simulink model "RUNES_demo"  (Simulink 7.4)
settings: Solver=ode45  StartTime=0.0  StopTime=inf  RelTol=1e-3
InitFcn:
  | init
values from neighbouring files (symbols this model uses):
  D = 30    [init.m]
  nbrOfMotes = 3    [init.m]
  R1 = 3    [init.m]
  R2 = 3    [init.m]
  trackLength = 800    [init.m]
  trackWidth = 200    [init.m]
undefined symbols (not defined in the file or in its folder): nodeXpos, nodeYpos, WLAN
libraries: truetime x14, simulink x6
settings Model: Creator=anton  LastModifiedBy=anton  ExtModeAutoUpdateStatusClock=off
settings DataIOCC: LimitDataPoints=off  SaveOutput=off  SaveTime=off
settings OptimizationCC: BooleanDataType=off
settings DebuggingCC: SaveWithParameterizedLinksMsg=none  SignalResolutionControl=TryResolveAllWithWarning  SolverPrmCheckMsg=none  MultiTaskDSMMsg=warning  MultiTaskCondExecSysMsg=none  UnconnectedInputMsg=none  UnconnectedOutputMsg=none  UnconnectedLineMsg=none  StrictBusMsg=None
settings HardwareCC: TargetUnknown=on
settings RTWCC: IncludeERTFirstTime=on

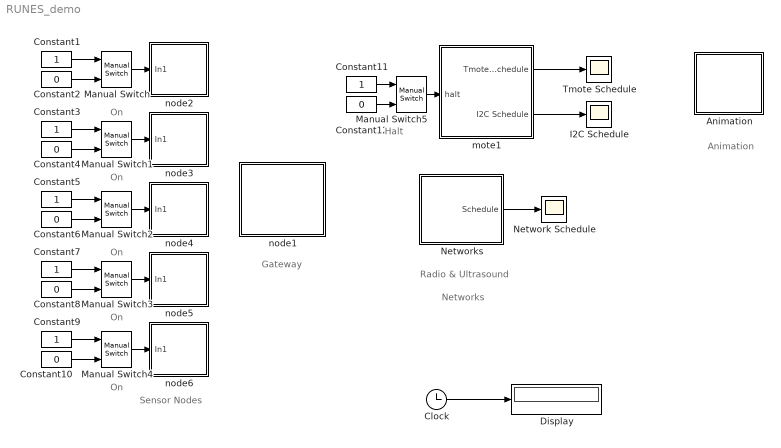
== system RUNES_demo ==
  note: Sensor Nodes
  note: Gateway
  note: Radio & Ultrasound
  note: Networks
  note: On
  note: On
  note: On
  note: On
  note: On
  note: Animation
  note: Halt
  Animation : Subsystem
  Clock : Clock
      settings: Decimation=10
  Constant{1,3,5,7,9,11} (6 alike) : Constant
  Constant{2,4,6,8,10,12} (6 alike) : Constant  Value=0
  Display : Display
  I2C Schedule : Scope
      settings: TimeRange=5  YMin=1  YMax=5.5  SaveName=nschedule1
  Manual Switch{,1..5} (6 alike) : simulink/Signal Routing/Manual Switch  SystemSampleTime=-1  sw=1  action=0  varsize=off
  Network Schedule : Scope
      settings: TimeRange=5  YMin=1  YMax=9  SaveName=nschedule
  Networks : Subsystem
  Tmote Schedule : Scope
      settings: TimeRange=5  YMin=1  YMax=9  SaveName=nschedule2
  mote1 : Subsystem  mask{moteNbr=1}
      mask Display: image(imread('RBBot.jpg'))
  node1 : Subsystem  mask{nodeNbr=1}
      mask init:
      | set_param(strcat(gcb,'/Goto'),'GotoTag',strcat('node',num2str(nodeNbr)));
      | set_param(strcat(gcb,'/X'),'Value',strcat('nodeXpos(',strcat(num2str(nodeNbr), ')')));
      | set_param(strcat(gcb,'/Y'),'Value',strcat('nodeYpos(',strcat(num2str(nodeNbr), ')')));
      mask Display: image(imread('gateway.jpg'))
  node2 : Subsystem  mask{nodeNbr=2}
      mask init: same as RUNES_demo/node1
      mask Display: image(imread('mote.jpg'))
  node3 : Subsystem  mask{nodeNbr=3}
      mask init: same as RUNES_demo/node1
      mask Display: image(imread('mote.jpg'))
  node4 : Subsystem  mask{nodeNbr=4}
      mask init: same as RUNES_demo/node1
      mask Display: image(imread('mote.jpg'))
  node5 : Subsystem  mask{nodeNbr=5}
      mask init: same as RUNES_demo/node1
      mask Display: image(imread('mote.jpg'))
  node6 : Subsystem  mask{nodeNbr=6}
      mask init: same as RUNES_demo/node1
      mask Display: image(imread('mote.jpg'))
  wires:
  Constant1/1 -> Manual Switch/1
  Constant2/1 -> Manual Switch/2
  Constant3/1 -> Manual Switch1/1
  Constant4/1 -> Manual Switch1/2
  Constant5/1 -> Manual Switch2/1
  Constant6/1 -> Manual Switch2/2
  Constant7/1 -> Manual Switch3/1
  Constant8/1 -> Manual Switch3/2
  Constant9/1 -> Manual Switch4/1
  Constant10/1 -> Manual Switch4/2
  Manual Switch/1 -> node2/1(In1)
  Manual Switch3/1 -> node5/1(In1)
  Manual Switch4/1 -> node6/1(In1)
  Manual Switch1/1 -> node3/1(In1)
  Networks/1(Schedule) -> Network Schedule/1
  Constant11/1 -> Manual Switch5/1
  Constant12/1 -> Manual Switch5/2
  Manual Switch5/1 -> mote1/1(halt)
  mote1/1(Tmote Schedule) -> Tmote Schedule/1
  mote1/2(I2C Schedule) -> I2C Schedule/1
  Clock/1 -> Display/1
  Manual Switch2/1 -> node4/1(In1)

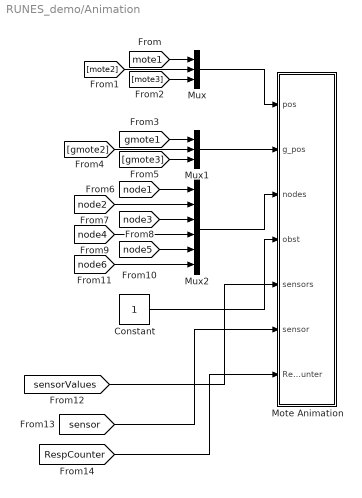
== system RUNES_demo/Animation ==
  Constant : Constant
  Mote Animation : Subsystem  mask{numMotes=nbrOfMotes, xmax=trackLength, ymax=trackWidth, ts=0.1}
      mask prompts: numMotes "Number of Motes"; ts "Update period"
  Mux : Mux  Inputs=[3 3 3]
  Mux1 : Mux  Inputs=[3 3 3]
  Mux2 : Mux  Inputs=6
  wires:
  Mux/1 -> Mote Animation/1(pos)
  [mote1] -> Mux/1
  [mote2] -> Mux/2
  [mote3] -> Mux/3
  Mux1/1 -> Mote Animation/2(g_pos)
  [gmote1] -> Mux1/1
  [gmote2] -> Mux1/2
  [gmote3] -> Mux1/3
  Constant/1 -> Mote Animation/4(obst)
  Mux2/1 -> Mote Animation/3(nodes)
  [node1] -> Mux2/1
  [node2] -> Mux2/2
  [node3] -> Mux2/3
  [node4] -> Mux2/4
  [node5] -> Mux2/5
  [node6] -> Mux2/6
  [sensorValues] -> Mote Animation/5(sensors)
  [sensor] -> Mote Animation/6(sensor)
  [RespCounter] -> Mote Animation/7(RespCounter)

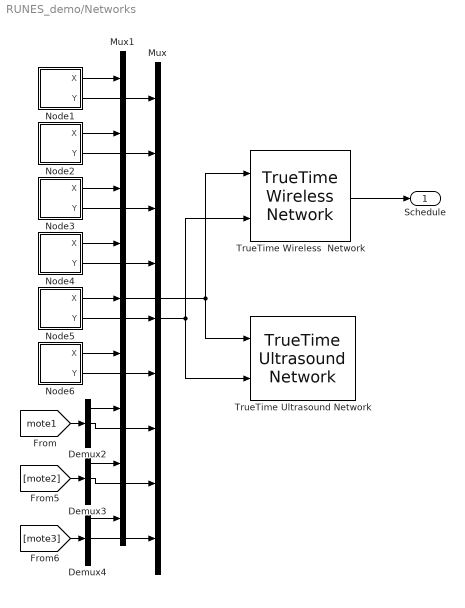
== system RUNES_demo/Networks ==
  Demux2 : Demux  Outputs=3
  Demux3 : Demux  Outputs=3
  Demux4 : Demux  Outputs=3
  Mux : Mux  Inputs=9
  Mux1 : Mux  Inputs=9
  Node1 : Subsystem  mask{nodeNbr=1}
      mask init:
      | set_param(strcat(gcb,'/From'),'GotoTag',strcat('node',num2str(nodeNbr)));
  Node2 : Subsystem  mask{nodeNbr=2}
      mask init:
      | set_param(strcat(gcb,'/From'),'GotoTag',strcat('node',num2str(nodeNbr)));
  Node3 : Subsystem  mask{nodeNbr=3}
      mask init:
      | set_param(strcat(gcb,'/From'),'GotoTag',strcat('node',num2str(nodeNbr)));
  Node4 : Subsystem  mask{nodeNbr=4}
      mask init:
      | set_param(strcat(gcb,'/From'),'GotoTag',strcat('node',num2str(nodeNbr)));
  Node5 : Subsystem  mask{nodeNbr=5}
      mask init:
      | set_param(strcat(gcb,'/From'),'GotoTag',strcat('node',num2str(nodeNbr)));
  Node6 : Subsystem  mask{nodeNbr=6}
      mask init:
      | set_param(strcat(gcb,'/From'),'GotoTag',strcat('node',num2str(nodeNbr)));
  TrueTime Ultrasound Network : truetime/TrueTime Ultrasound Network  SystemSampleTime=-1  nwnbr=2  nnodes=9  reach=260  pinglength=0.0  speedofsound=34400.0  scheduleoutput=off
  TrueTime Wireless  Network : truetime/TrueTime Wireless  Network  SystemSampleTime=-1  nwtype=802.11b (WLAN)  nwnbr=1  nnodes=9  rate=250000  minsize=248  transpower=transmitPower  threshold=receiverThreshold  use_pathloss_function=default  pathloss=pathloss  acktimeout=0.000864  retrylimit=3  error_threshold=errorCodingThreshold  lossprob=0  seed=0  scheduleoutput=on  poweroutput=off
  Schedule : Outport
  wires:
  Node1/1(X) -> Mux1/1
  Node2/1(X) -> Mux1/2
  Node3/1(X) -> Mux1/3
  Node4/1(X) -> Mux1/4
  Node5/1(X) -> Mux1/5
  Node6/1(X) -> Mux1/6
  Node6/2(Y) -> Mux/6
  Node5/2(Y) -> Mux/5
  Node4/2(Y) -> Mux/4
  Node3/2(Y) -> Mux/3
  Node2/2(Y) -> Mux/2
  Node1/2(Y) -> Mux/1
  [mote1] -> Demux2/1
  Demux2/1 -> Mux1/7
  [mote2] -> Demux3/1
  Demux3/1 -> Mux1/8
  Demux3/2 -> Mux/8
  Demux2/2 -> Mux/7
  [mote3] -> Demux4/1
  Demux4/1 -> Mux1/9
  Demux4/2 -> Mux/9
  Mux1/1 -> TrueTime Wireless  Network/1, TrueTime Ultrasound Network/1
  Mux/1 -> TrueTime Ultrasound Network/2, TrueTime Wireless  Network/2
  TrueTime Wireless  Network/1 -> Schedule/1

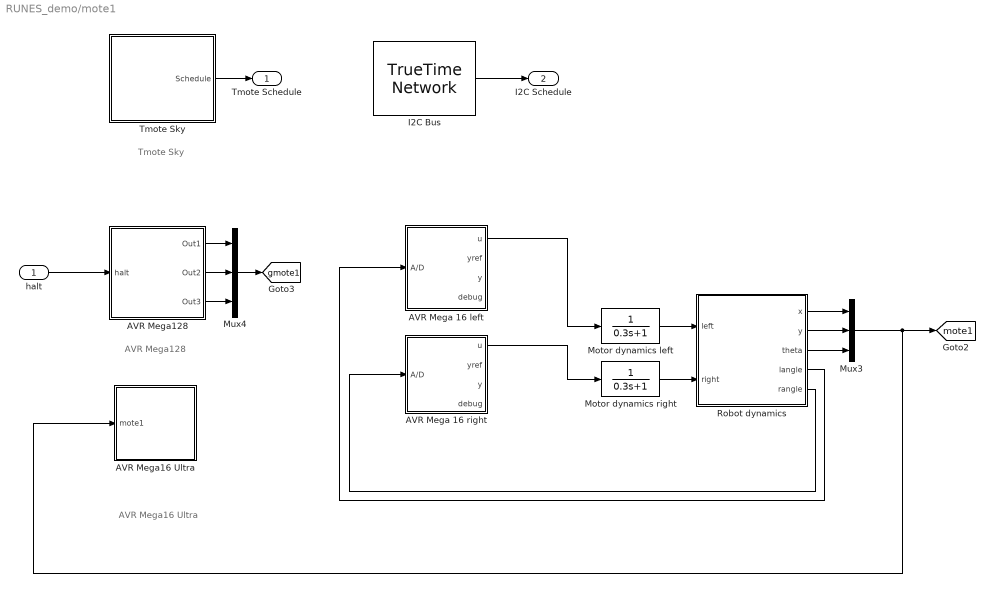
== system RUNES_demo/mote1 ==
  note: Tmote Sky
  note: AVR Mega16 Ultra
  note: AVR Mega128
  halt : Inport
  AVR Mega 16 left : Subsystem
      mask Display: image(imread('mega16.jpg'))
  AVR Mega 16 right : Subsystem
      mask Display: image(imread('mega16.jpg'))
  AVR Mega128 : Subsystem
      mask Display: image(imread('mega128.jpg'))
  AVR Mega16 Ultra : Subsystem
      mask Display: image(imread('mega16.jpg'))
  I2C Bus : truetime/TrueTime Network  SystemSampleTime=-1  nwtype=CSMA/CD (Ethernet)  nwnbr=3  nnodes=5  rate=10000000  minsize=512  lossprob=0  seed=0  bandwidths=[0.5 0.5]  slotsize=512  schedule=[1 1 2]  memsize=80000  buftype=Common buffer  overflow=Retransmit  dynSchedule=0  miniSlotSize=0  NIT=0  QSortMode=FIFO  sync=0  irtSchedule=0  nrtLength=0  nodeGraph=0  scheduleoutput=on
  Motor dynamics left : TransferFcn  Denominator=[0.3 1]
  Motor dynamics right : TransferFcn  Denominator=[0.3 1]
  Mux3 : Mux  Inputs=3
  Mux4 : Mux  Inputs=3
  Robot dynamics : Subsystem  TreatAsAtomicUnit=on
      mask Display: image(imread('model.png'))
  Tmote Sky : Subsystem
      mask Display: image(imread('Tmote.jpg'))
  Tmote Schedule : Outport
  I2C Schedule : Outport  Port=2
  tag scope: gmote1=global, mote1=global
  wires:
  Tmote Sky/1(Schedule) -> Tmote Schedule/1
  I2C Bus/1 -> I2C Schedule/1
  Mux4/1 -> [gmote1]
  halt/1 -> AVR Mega128/1(halt)
  Robot dynamics/4(langle) -> AVR Mega 16 left/1(A/D)
  Robot dynamics/5(rangle) -> AVR Mega 16 right/1(A/D)
  Motor dynamics right/1 -> Robot dynamics/2(right)
  Motor dynamics left/1 -> Robot dynamics/1(left)
  AVR Mega 16 left/1(u) -> Motor dynamics left/1
  AVR Mega 16 right/1(u) -> Motor dynamics right/1
  AVR Mega128/3(Out3) -> Mux4/3
  AVR Mega128/2(Out2) -> Mux4/2
  AVR Mega128/1(Out1) -> Mux4/1
  Robot dynamics/1(x) -> Mux3/1
  Robot dynamics/2(y) -> Mux3/2
  Robot dynamics/3(theta) -> Mux3/3
  Mux3/1 -> [mote1], AVR Mega16 Ultra/1(mote1)

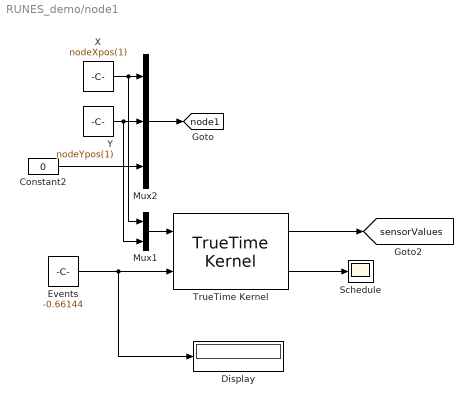
== system RUNES_demo/node1 ==
  Constant2 : Constant  Value=0
  Display : Display
  Events : Constant  Value=-0.66144
  Mux1 : Mux  Inputs=2
  Mux2 : Mux  Inputs=3
  Schedule : Scope
      settings: TickLabels=on  TimeRange=3.5  YMin=0  YMax=9.5  DataFormat=Array
  TrueTime Kernel : truetime/TrueTime Kernel  SystemSampleTime=-1  sfun=node_init  args=nodeNbr  ninputsoutputs=[2 5]  ntriggers=1  trigtype=falling  nwnodenbr=[1 nodeNbr; 2 nodeNbr]  clockoffsetdrift=[0 0]  schedoutput=on  battery=off  poweroutput=off  label=1: 1\n2: 1
  X : Constant  Value=nodeXpos(1)
  Y : Constant  Value=nodeYpos(1)
  tag scope: node1=global, sensorValues=global
  wires:
  X/1 -> Mux2/1, Mux1/1
  Y/1 -> Mux2/2, Mux1/2
  Mux2/1 -> [node1]
  Constant2/1 -> Mux2/3
  TrueTime Kernel/1 -> [sensorValues]
  Mux1/1 -> TrueTime Kernel/1
  TrueTime Kernel/2 -> Schedule/1
  Events/1 -> Display/1, TrueTime Kernel/2

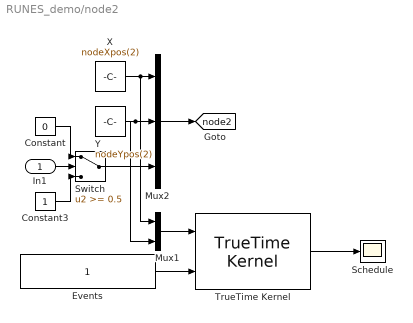
== system RUNES_demo/node2 ==
  In1 : Inport
  Constant : Constant  Value=0
  Constant3 : Constant
  Events : Constant
  Mux1 : Mux  Inputs=2
  Mux2 : Mux  Inputs=3
  Schedule : Scope
      settings: TickLabels=on  TimeRange=3.5  YMin=1.8  YMax=3.7  DataFormat=Array
  Switch : Switch  Threshold=0.5  SaturateOnIntegerOverflow=on  InputSameDT=on
  TrueTime Kernel : truetime/TrueTime Kernel  SystemSampleTime=-1  sfun=node_init  args=nodeNbr  ninputsoutputs=[2 0]  ntriggers=1  trigtype=either  nwnodenbr=[1 nodeNbr; 2 nodeNbr]  clockoffsetdrift=[0 0]  schedoutput=on  battery=off  poweroutput=off  label=1: 2\n2: 2
  X : Constant  Value=nodeXpos(2)
  Y : Constant  Value=nodeYpos(2)
  tag scope: node2=global
  wires:
  TrueTime Kernel/1 -> Schedule/1
  Events/1 -> TrueTime Kernel/2
  Mux2/1 -> [node2]
  Switch/1 -> Mux2/3
  Y/1 -> Mux1/2, Mux2/2
  X/1 -> Mux1/1, Mux2/1
  In1/1 -> Switch/2
  Constant3/1 -> Switch/3
  Constant/1 -> Switch/1
  Mux1/1 -> TrueTime Kernel/1

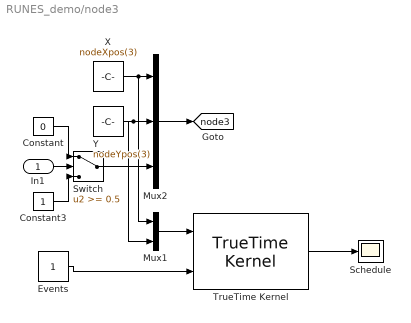
== system RUNES_demo/node3 ==
  In1 : Inport
  Constant : Constant  Value=0
  Constant3 : Constant
  Events : Constant
  Mux1 : Mux  Inputs=2
  Mux2 : Mux  Inputs=3
  Schedule : Scope
      settings: TickLabels=on  TimeRange=3.5  YMin=1.8  YMax=3.7  DataFormat=Array
  Switch : Switch  Threshold=0.5  SaturateOnIntegerOverflow=on  InputSameDT=on
  TrueTime Kernel : truetime/TrueTime Kernel  SystemSampleTime=-1  sfun=node_init  args=nodeNbr  ninputsoutputs=[2 0]  ntriggers=1  trigtype=either  nwnodenbr=[1 nodeNbr; 2 nodeNbr]  clockoffsetdrift=[0 0]  schedoutput=on  battery=off  poweroutput=off  label=1: 3\n2: 3
  X : Constant  Value=nodeXpos(3)
  Y : Constant  Value=nodeYpos(3)
  tag scope: node3=global
  wires:
  Mux1/1 -> TrueTime Kernel/1
  Constant/1 -> Switch/1
  Constant3/1 -> Switch/3
  In1/1 -> Switch/2
  X/1 -> Mux2/1, Mux1/1
  Y/1 -> Mux2/2, Mux1/2
  Switch/1 -> Mux2/3
  Mux2/1 -> [node3]
  Events/1 -> TrueTime Kernel/2
  TrueTime Kernel/1 -> Schedule/1

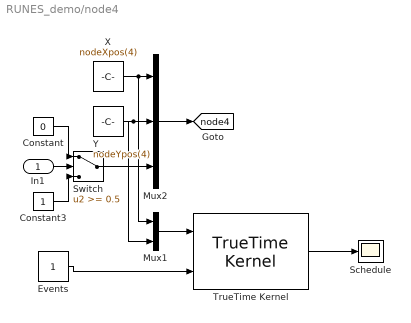
== system RUNES_demo/node4 ==
  In1 : Inport
  Constant : Constant  Value=0
  Constant3 : Constant
  Events : Constant
  Mux1 : Mux  Inputs=2
  Mux2 : Mux  Inputs=3
  Schedule : Scope
      settings: TickLabels=on  TimeRange=3.5  YMin=1.8  YMax=3.7  DataFormat=Array
  Switch : Switch  Threshold=0.5  SaturateOnIntegerOverflow=on  InputSameDT=on
  TrueTime Kernel : truetime/TrueTime Kernel  SystemSampleTime=-1  sfun=node_init  args=nodeNbr  ninputsoutputs=[2 0]  ntriggers=1  trigtype=either  nwnodenbr=[1 nodeNbr; 2 nodeNbr]  clockoffsetdrift=[0 0]  schedoutput=on  battery=off  poweroutput=off  label=1: 4\n2: 4
  X : Constant  Value=nodeXpos(4)
  Y : Constant  Value=nodeYpos(4)
  tag scope: node4=global
  wires:
  TrueTime Kernel/1 -> Schedule/1
  Events/1 -> TrueTime Kernel/2
  Mux2/1 -> [node4]
  Switch/1 -> Mux2/3
  Y/1 -> Mux1/2, Mux2/2
  X/1 -> Mux1/1, Mux2/1
  In1/1 -> Switch/2
  Constant3/1 -> Switch/3
  Constant/1 -> Switch/1
  Mux1/1 -> TrueTime Kernel/1

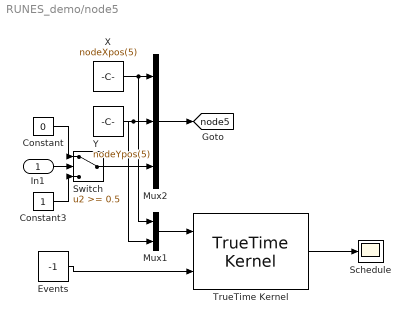
== system RUNES_demo/node5 ==
  In1 : Inport
  Constant : Constant  Value=0
  Constant3 : Constant
  Events : Constant  Value=-1
  Mux1 : Mux  Inputs=2
  Mux2 : Mux  Inputs=3
  Schedule : Scope
      settings: TickLabels=on  TimeRange=3.5  YMin=1.8  YMax=3.7  DataFormat=Array
  Switch : Switch  Threshold=0.5  SaturateOnIntegerOverflow=on  InputSameDT=on
  TrueTime Kernel : truetime/TrueTime Kernel  SystemSampleTime=-1  sfun=node_init  args=nodeNbr  ninputsoutputs=[2 0]  ntriggers=1  trigtype=either  nwnodenbr=[1 nodeNbr; 2 nodeNbr]  clockoffsetdrift=[0 0]  schedoutput=on  battery=off  poweroutput=off  label=1: 5\n2: 5
  X : Constant  Value=nodeXpos(5)
  Y : Constant  Value=nodeYpos(5)
  tag scope: node5=global
  wires:
  Mux1/1 -> TrueTime Kernel/1
  Constant/1 -> Switch/1
  Constant3/1 -> Switch/3
  In1/1 -> Switch/2
  X/1 -> Mux2/1, Mux1/1
  Y/1 -> Mux2/2, Mux1/2
  Switch/1 -> Mux2/3
  Mux2/1 -> [node5]
  Events/1 -> TrueTime Kernel/2
  TrueTime Kernel/1 -> Schedule/1

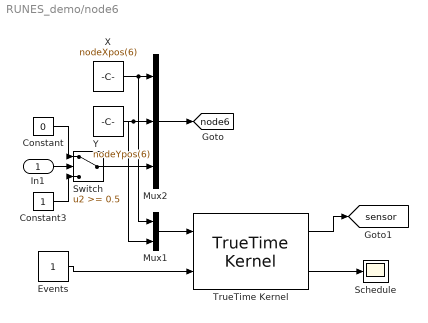
== system RUNES_demo/node6 ==
  In1 : Inport
  Constant : Constant  Value=0
  Constant3 : Constant
  Events : Constant
  Mux1 : Mux  Inputs=2
  Mux2 : Mux  Inputs=3
  Schedule : Scope
      settings: TickLabels=on  TimeRange=3.5  YMin=1.8  YMax=3.7  DataFormat=Array
  Switch : Switch  Threshold=0.5  SaturateOnIntegerOverflow=on  InputSameDT=on
  TrueTime Kernel : truetime/TrueTime Kernel  SystemSampleTime=-1  sfun=node_init  args=nodeNbr  ninputsoutputs=[2 1]  ntriggers=1  trigtype=either  nwnodenbr=[1 nodeNbr; 2 nodeNbr]  clockoffsetdrift=[0 0]  schedoutput=on  battery=off  poweroutput=off  label=1: 6\n2: 6
  X : Constant  Value=nodeXpos(6)
  Y : Constant  Value=nodeYpos(6)
  tag scope: node6=global, sensor=global
  wires:
  TrueTime Kernel/2 -> Schedule/1
  Events/1 -> TrueTime Kernel/2
  Mux2/1 -> [node6]
  Switch/1 -> Mux2/3
  Y/1 -> Mux1/2, Mux2/2
  X/1 -> Mux1/1, Mux2/1
  In1/1 -> Switch/2
  Constant3/1 -> Switch/3
  Constant/1 -> Switch/1
  Mux1/1 -> TrueTime Kernel/1
  TrueTime Kernel/1 -> [sensor]

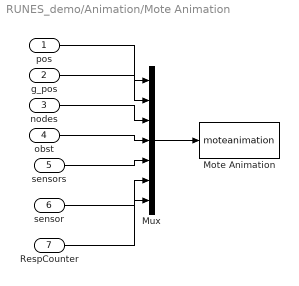
== system RUNES_demo/Animation/Mote Animation ==
  pos : Inport
  g_pos : Inport  Port=2
  nodes : Inport  Port=3
  obst : Inport  Port=4
  sensors : Inport  Port=5
  sensor : Inport  Port=6
  RespCounter : Inport  Port=7
  Mote Animation : S-Function  FunctionName=moteanimation  Parameters=[numMotes ts xmax ymax]  EnableBusSupport=off
      settings: DeleteFcn=if ~isempty(findobj('type','figure','name','dblpend1 Animation'));close('dblpend1 Animation'); end;
  Mux : Mux  Inputs=7
  wires:
  pos/1 -> Mux/1
  g_pos/1 -> Mux/2
  nodes/1 -> Mux/3
  obst/1 -> Mux/4
  Mux/1 -> Mote Animation/1
  sensors/1 -> Mux/5
  sensor/1 -> Mux/6
  RespCounter/1 -> Mux/7

== system RUNES_demo/Networks/Node1 ==
  Add : Sum  InputSameDT=on  OutDataTypeStr=Inherit: Same as first input
  Add1 : Sum  InputSameDT=on  OutDataTypeStr=Inherit: Same as first input
  Demux1 : Demux  Outputs=3
  FarAway : Constant  Value=999999999
  Product : Product  RndMeth=Zero  InputSameDT=on  OutDataTypeStr=Inherit: Same as first input
  X : Outport
  Y : Outport  Port=2
  wires:
  [node1] -> Demux1/1
  Add/1 -> X/1
  Add1/1 -> Y/1
  Demux1/1 -> Add/1
  Demux1/2 -> Add1/1
  FarAway/1 -> Product/2
  Product/1 -> Add/2, Add1/2
  Demux1/3 -> Product/1

== system RUNES_demo/Networks/Node2 ==
  Add : Sum  InputSameDT=on  OutDataTypeStr=Inherit: Same as first input
  Add1 : Sum  InputSameDT=on  OutDataTypeStr=Inherit: Same as first input
  Demux1 : Demux  Outputs=3
  FarAway : Constant  Value=999999999
  Product : Product  RndMeth=Zero  InputSameDT=on  OutDataTypeStr=Inherit: Same as first input
  X : Outport
  Y : Outport  Port=2
  wires:
  Product/1 -> Add1/2, Add/2
  Demux1/3 -> Product/1
  FarAway/1 -> Product/2
  Demux1/2 -> Add1/1
  Demux1/1 -> Add/1
  Add1/1 -> Y/1
  Add/1 -> X/1
  [node2] -> Demux1/1

== system RUNES_demo/Networks/Node3 ==
  Add : Sum  InputSameDT=on  OutDataTypeStr=Inherit: Same as first input
  Add1 : Sum  InputSameDT=on  OutDataTypeStr=Inherit: Same as first input
  Demux1 : Demux  Outputs=3
  FarAway : Constant  Value=999999999
  Product : Product  RndMeth=Zero  InputSameDT=on  OutDataTypeStr=Inherit: Same as first input
  X : Outport
  Y : Outport  Port=2
  wires:
  [node3] -> Demux1/1
  Add/1 -> X/1
  Add1/1 -> Y/1
  Demux1/1 -> Add/1
  Demux1/2 -> Add1/1
  FarAway/1 -> Product/2
  Demux1/3 -> Product/1
  Product/1 -> Add/2, Add1/2

== system RUNES_demo/Networks/Node4 ==
  Add : Sum  InputSameDT=on  OutDataTypeStr=Inherit: Same as first input
  Add1 : Sum  InputSameDT=on  OutDataTypeStr=Inherit: Same as first input
  Demux1 : Demux  Outputs=3
  FarAway : Constant  Value=999999999
  Product : Product  RndMeth=Zero  InputSameDT=on  OutDataTypeStr=Inherit: Same as first input
  X : Outport
  Y : Outport  Port=2
  wires:
  Product/1 -> Add1/2, Add/2
  Demux1/3 -> Product/1
  FarAway/1 -> Product/2
  Demux1/2 -> Add1/1
  Demux1/1 -> Add/1
  Add1/1 -> Y/1
  Add/1 -> X/1
  [node4] -> Demux1/1

== system RUNES_demo/Networks/Node5 ==
  Add : Sum  InputSameDT=on  OutDataTypeStr=Inherit: Same as first input
  Add1 : Sum  InputSameDT=on  OutDataTypeStr=Inherit: Same as first input
  Demux1 : Demux  Outputs=3
  FarAway : Constant  Value=999999999
  Product : Product  RndMeth=Zero  InputSameDT=on  OutDataTypeStr=Inherit: Same as first input
  X : Outport
  Y : Outport  Port=2
  wires:
  [node5] -> Demux1/1
  Add/1 -> X/1
  Add1/1 -> Y/1
  Demux1/1 -> Add/1
  Demux1/2 -> Add1/1
  FarAway/1 -> Product/2
  Demux1/3 -> Product/1
  Product/1 -> Add/2, Add1/2

== system RUNES_demo/Networks/Node6 ==
  Add : Sum  InputSameDT=on  OutDataTypeStr=Inherit: Same as first input
  Add1 : Sum  InputSameDT=on  OutDataTypeStr=Inherit: Same as first input
  Demux1 : Demux  Outputs=3
  FarAway : Constant  Value=999999999
  Product : Product  RndMeth=Zero  InputSameDT=on  OutDataTypeStr=Inherit: Same as first input
  X : Outport
  Y : Outport  Port=2
  wires:
  Product/1 -> Add1/2, Add/2
  Demux1/3 -> Product/1
  FarAway/1 -> Product/2
  Demux1/2 -> Add1/1
  Demux1/1 -> Add/1
  Add1/1 -> Y/1
  Add/1 -> X/1
  [node6] -> Demux1/1

== system RUNES_demo/mote1/AVR Mega 16 left ==
  A/D : Inport
  AVR Mega 16-left : truetime/TrueTime Kernel  SystemSampleTime=-1  sfun=left_init  args=1  ninputsoutputs=[1 4]  ntriggers=0  trigtype=falling  nwnodenbr=[3 2]  clockoffsetdrift=[0 0]  schedoutput=off  battery=off  poweroutput=off  label=3: 2
  Demux : Demux
  u : Outport
  yref : Outport  Port=2
  y : Outport  Port=3
  debug : Outport  Port=4
  wires:
  AVR Mega 16-left/1 -> Demux/1
  Demux/1 -> u/1
  Demux/2 -> yref/1
  Demux/3 -> y/1
  Demux/4 -> debug/1
  A/D/1 -> AVR Mega 16-left/1

== system RUNES_demo/mote1/AVR Mega 16 right ==
  A/D : Inport
  AVR Mega 16-left : truetime/TrueTime Kernel  SystemSampleTime=-1  sfun=right_init  args=1  ninputsoutputs=[1 4]  ntriggers=0  trigtype=falling  nwnodenbr=[3 3]  clockoffsetdrift=[0 0]  schedoutput=off  battery=off  poweroutput=off  label=3: 3
  Demux : Demux
  u : Outport
  yref : Outport  Port=2
  y : Outport  Port=3
  debug : Outport  Port=4
  wires:
  A/D/1 -> AVR Mega 16-left/1
  Demux/4 -> debug/1
  Demux/3 -> y/1
  Demux/2 -> yref/1
  Demux/1 -> u/1
  AVR Mega 16-left/1 -> Demux/1

== system RUNES_demo/mote1/AVR Mega128 ==
  halt : Inport
  AVR Mega 128 : truetime/TrueTime Kernel  SystemSampleTime=-1  sfun=mega128_init  args=1  ninputsoutputs=[1 3]  ntriggers=0  trigtype=falling  nwnodenbr=[3 4]  clockoffsetdrift=[0 0]  schedoutput=off  battery=off  poweroutput=off  label=3: 4
  Demux : Demux  Outputs=3
  Out1 : Outport
  Out2 : Outport  Port=2
  Out3 : Outport  Port=3
  wires:
  Demux/1 -> Out1/1
  Demux/2 -> Out2/1
  Demux/3 -> Out3/1
  AVR Mega 128/1 -> Demux/1
  halt/1 -> AVR Mega 128/1

== system RUNES_demo/mote1/AVR Mega16 Ultra ==
  mote1 : Inport
  AVR Mega16 Ultra : truetime/TrueTime Kernel  SystemSampleTime=-1  sfun=megaultra_init  args=1  ninputsoutputs=[3 1]  ntriggers=0  trigtype=falling  nwnodenbr=[2 7; 3 5]  clockoffsetdrift=[0 0]  schedoutput=off  battery=off  poweroutput=off  label=2: 7\n3: 5
  wires:
  mote1/1 -> AVR Mega16 Ultra/1

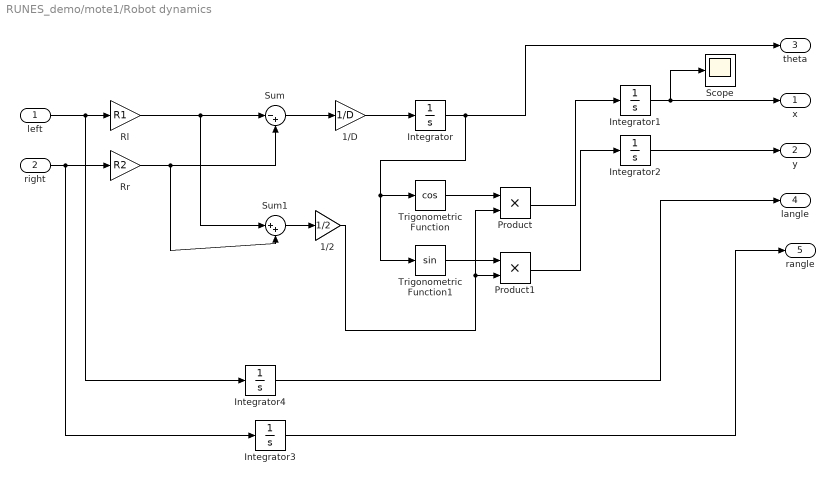
== system RUNES_demo/mote1/Robot dynamics ==
  left : Inport
  right : Inport  Port=2
  1/2 : Gain  Gain=1/2  OutDataTypeStr=Inherit: Same as input  ParamDataTypeStr=Inherit: Same as input
  1/D : Gain  Gain=1/D  OutDataTypeStr=Inherit: Same as input  ParamDataTypeStr=Inherit: Same as input
  Integrator{,1..4} (5 alike) : Integrator
  Product : Product  RndMeth=Zero  InputSameDT=on  OutDataTypeStr=Inherit: Same as first input
  Product1 : Product  RndMeth=Zero  InputSameDT=on  OutDataTypeStr=Inherit: Same as first input
  Rl : Gain  Gain=R1  OutDataTypeStr=Inherit: Same as input  ParamDataTypeStr=Inherit: Same as input
  Rr : Gain  Gain=R2  OutDataTypeStr=Inherit: Same as input  ParamDataTypeStr=Inherit: Same as input
  Scope : Scope
      settings: TimeRange=100  YMin=0  YMax=550  SaveName=ScopeData3
  Sum : Sum  Inputs=|-+  InputSameDT=on  OutDataTypeStr=Inherit: Same as first input
  Sum1 : Sum  Inputs=|++  InputSameDT=on  OutDataTypeStr=Inherit: Same as first input
  Trigonometric Function : Trigonometry  Operator=cos
  Trigonometric Function1 : Trigonometry
  x : Outport
  y : Outport  Port=2
  theta : Outport  Port=3
  langle : Outport  Port=4
  rangle : Outport  Port=5
  wires:
  left/1 -> Rl/1, Integrator4/1
  right/1 -> Rr/1, Integrator3/1
  Rl/1 -> Sum/1, Sum1/1
  Rr/1 -> Sum/2, Sum1/2
  Sum/1 -> 1/D/1
  1/D/1 -> Integrator/1
  Integrator/1 -> Trigonometric Function/1, Trigonometric Function1/1, theta/1
  Trigonometric Function/1 -> Product/1
  Trigonometric Function1/1 -> Product1/1
  Sum1/1 -> 1/2/1
  Product/1 -> Integrator1/1
  Product1/1 -> Integrator2/1
  Integrator1/1 -> x/1, Scope/1
  Integrator2/1 -> y/1
  Integrator4/1 -> langle/1
  Integrator3/1 -> rangle/1
  1/2/1 -> Product1/2, Product/2

== system RUNES_demo/mote1/Tmote Sky ==
  Events : Constant
  TrueTime Kernel : truetime/TrueTime Kernel  SystemSampleTime=-1  sfun=tmote_init  args=1  ninputsoutputs=[1 1]  ntriggers=1  trigtype=falling  nwnodenbr=[1 7; 3 1]  clockoffsetdrift=[0 0]  schedoutput=on  battery=off  poweroutput=off  label=1: 7\n3: 1
  Schedule : Outport
  tag scope: RespCounter=global
  wires:
  TrueTime Kernel/2 -> Schedule/1
  TrueTime Kernel/1 -> [RespCounter]
  Events/1 -> TrueTime Kernel/2
